simulink model "clase07012021"  (R2020b)
settings: Solver=VariableStepAuto  StartTime=0.0  StopTime=1  RelTol=1e-3
libraries: commutil2 x1, commdigbbndpm3 x1
settings Model: Creator=fernando  LastModifiedBy=fernando

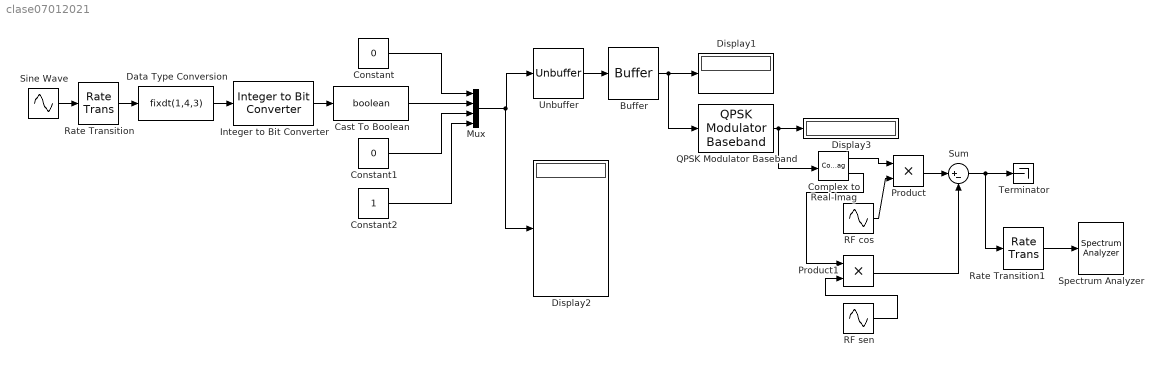
== system clase07012021 ==
  Buffer : Buffer  N=2  OutputFrames=off
  Cast To Boolean : DataTypeConversion  OutDataTypeStr=boolean
  Complex to Real-Imag : ComplexToRealImag
  Constant : Constant  Value=0  OutDataTypeStr=boolean
  Constant1 : Constant  Value=0  OutDataTypeStr=boolean
  Constant2 : Constant  OutDataTypeStr=boolean
  Data Type Conversion : DataTypeConversion  OutDataTypeStr=fixdt(1,4,3)
  Display1 : Display
  Display2 : Display
  Display3 : Display
  Integer to Bit Converter : commutil2/Integer to Bit Converter  nbits=4  signedInputValues=Unsigned  bitOrder=MSB first  outDtype=Inherit via internal rule
  Mux : Mux
  Product : Product
  Product1 : Product
  QPSK Modulator Baseband : commdigbbndpm3/QPSK Modulator Baseband  InType=Bit  Enc=Gray  Ph=pi/4  outDtype=double  outWordLen=16  outUDDataType=sfix(16)  outFracLenMode=Best precision  outFracLen=15  outDataTypeStr=double  outLastDataTypeStr=double
      settings: SourceProductName=Communications Toolbox
  RF cos : Sin  Frequency=2*pi/2  SampleTime=0
  RF sen : Sin  Frequency=2*pi*400  SampleTime=0
  Rate Transition : RateTransition  OutPortSampleTime=1/4000
  Rate Transition1 : RateTransition  OutPortSampleTime=1/2e6
  Sine Wave : Sin  Frequency=2*pi*400  SampleTime=0
  Spectrum Analyzer : SpectrumAnalyzer
  Sum : Sum  Inputs=|+-
  Terminator : Terminator
  Unbuffer : Unbuffer
  wires:
  Constant2/1 -> Mux/4
  Rate Transition/1 -> Data Type Conversion/1
  Constant1/1 -> Mux/3
  Sine Wave/1 -> Rate Transition/1
  Data Type Conversion/1 -> Integer to Bit Converter/1
  Integer to Bit Converter/1 -> Cast To Boolean/1
  Mux/1 -> Display2/1, Unbuffer/1
  Constant/1 -> Mux/1
  Cast To Boolean/1 -> Mux/2
  QPSK Modulator Baseband/1 -> Display3/1, Complex to Real-Imag/1
  RF cos/1 -> Product/2
  Complex to Real-Imag/1 -> Product/1
  Complex to Real-Imag/2 -> Product1/1
  Rate Transition1/1 -> Spectrum Analyzer/1
  RF sen/1 -> Product1/2
  Product/1 -> Sum/1
  Product1/1 -> Sum/2
  Sum/1 -> Rate Transition1/1, Terminator/1
  Unbuffer/1 -> Buffer/1
  Buffer/1 -> QPSK Modulator Baseband/1, Display1/1
